simulink model "Part11_Unreal_Engine"  (R2021a)
settings: Solver=VariableStepAuto  StartTime=0.0  StopTime=100  RelTol=1e-3
libraries: vdynlib x3, vrlib x2, simulink x2, sim3dlib x1, mpcadaslib x1, pid_lib x1
settings Model: Creator=QZHAN112  LastModifiedBy=QZHAN112

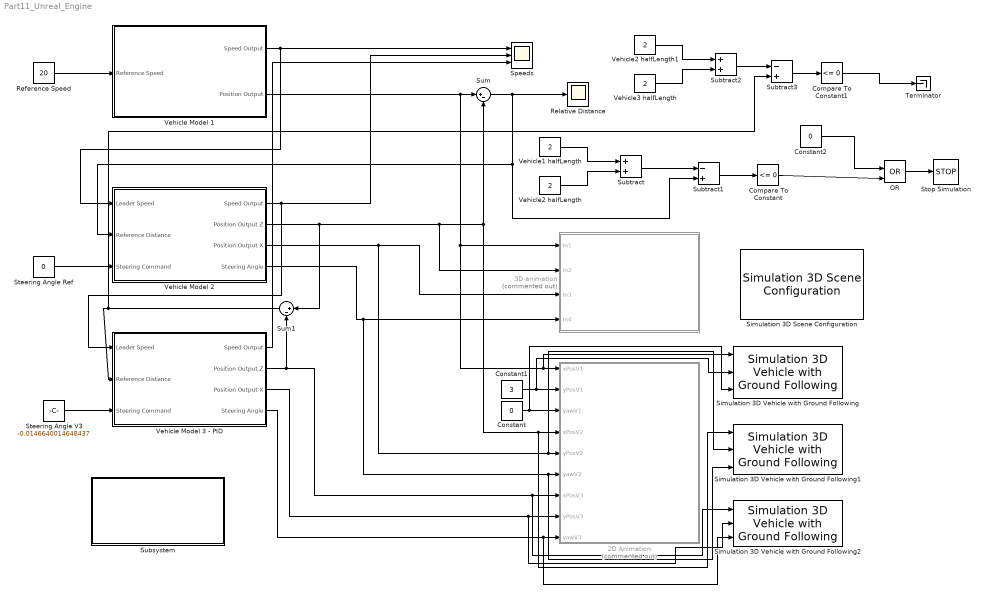
== system Part11_Unreal_Engine ==
  2D Animation : Subsystem  Commented=on
  3D animation : Subsystem  Commented=on
  Compare To Constant : simulink/Logic and Bit Operations/Compare To Constant  relop=<=  const=0  OutDataTypeStr=boolean
  Compare To Constant1 : simulink/Logic and Bit Operations/Compare To Constant  relop=<=  const=0  OutDataTypeStr=boolean
  Constant : Constant  Value=0
  Constant1 : Constant  Value=3
  Constant2 : Constant  Value=0
  OR : Logic  Operator=OR  IconShape=distinctive  AllPortsSameDT=off  OutDataTypeStr=boolean
  Reference Speed : Constant  Value=20
  Relative Distance : Scope
  Simulation 3D Scene Configuration : sim3dlib/Simulation 3D Scene Configuration  Priority=0  ProjectFormat=Default Scenes  SceneDesc=Straight road  ProjectName=C:\Program Files\MATLAB\R2021a\toolbox\shared\sim3d_projects\automotive_project\UE4\WindowsNoEditor\VehicleSimulation.exe  ScenePath=/Game/Maps/HwStrght  vehTagList={'Scene Origin';'SimulinkVehicle1';'SimulinkVehicle2';'SimulinkVehicle3'}  vehTag=SimulinkVehicle2  OpVisEn=off  Ts=0.1  EnableWindow=on  EnableWeather=off  SunAltitude=40.0  SunAzimuth=90  clouds=10  wind=1  fog=0  rain=0  sensorTag=MainCamera1  sensorId=1  sensorName=MainCamera1  mountLoc=Origin  offsetFlag=off  tmountOffset=[0, 0, 0]  rmountOffset=[0, 0, 0]  HorizontalResolution=1280  VerticalResolution=720  HorizontalFOV=60  mountPoint=[0 0 0]  mountOrientation=[0 0 0]  aMode=3  ID=1
      settings: SourceProductBaseCode=DR,UV,VE
  Simulation 3D Vehicle with Ground Following : vdynlib/Vehicle Scenarios/Sim3D/Sim3D Vehicle/Components/Simulation 3D Vehicle with Ground Following  Priority=-1  PassVehMesh=Small pickup truck  MeshPath=/MathWorksSimulation/Vehicles/Muscle/Meshes/SK_MuscleCar.SK_MuscleCar  TrackWidth=1.9  WheelBase=3  WheelRadius=0.35  VehColor=Red  InitialPos=[40, 0, 0]  InitialRot=[0, 0, 0]  ActorName=SimulinkVehicle1  VehLightsControl=off  HeadlightColor=[ 1, 1, 1 ]  HighBeamIntensity=100000  LowBeamIntensity=60000  HighBeamConeAngle=1.22  LowBeamConeAngle=1.22  LeftHeadlightOrientation=[ 0, 0 ]  RightHeadlightOrientation=[ 0, 0 ]  BrakelightIntensity=200  ReverselightIntensity=500  SignallightIntensity=500  SignallightPeriod=1  SignalPulseWidth=50  SampleTime=0.1  ActorType=SimulinkVehicle  ID=1  aMode=2  ActorTag=SimulinkVehicle1  CoordinateScheme=SAE
      settings: SourceProductBaseCode=VE
  Simulation 3D Vehicle with Ground Following1 : vdynlib/Vehicle Scenarios/Sim3D/Sim3D Vehicle/Components/Simulation 3D Vehicle with Ground Following  Priority=-1  PassVehMesh=Sedan  MeshPath=/MathWorksSimulation/Vehicles/Muscle/Meshes/SK_MuscleCar.SK_MuscleCar  TrackWidth=1.9  WheelBase=3  WheelRadius=0.35  VehColor=Silver  InitialPos=[20, 0, 0]  InitialRot=[0, 0, 0]  ActorName=SimulinkVehicle2  VehLightsControl=off  HeadlightColor=[ 1, 1, 1 ]  HighBeamIntensity=100000  LowBeamIntensity=60000  HighBeamConeAngle=1.22  LowBeamConeAngle=1.22  LeftHeadlightOrientation=[ 0, 0 ]  RightHeadlightOrientation=[ 0, 0 ]  BrakelightIntensity=200  ReverselightIntensity=500  SignallightIntensity=500  SignallightPeriod=1  SignalPulseWidth=50  SampleTime=0.1  ActorType=SimulinkVehicle  ID=2  aMode=2  ActorTag=SimulinkVehicle2  CoordinateScheme=SAE
      settings: SourceProductBaseCode=VE
  Simulation 3D Vehicle with Ground Following2 : vdynlib/Vehicle Scenarios/Sim3D/Sim3D Vehicle/Components/Simulation 3D Vehicle with Ground Following  Priority=-1  PassVehMesh=Box truck  MeshPath=/MathWorksSimulation/Vehicles/Muscle/Meshes/SK_MuscleCar.SK_MuscleCar  TrackWidth=1.9  WheelBase=3  WheelRadius=0.35  VehColor=Green  InitialPos=[0, 100, 0]  InitialRot=[0, 0, 0]  ActorName=SimulinkVehicle3  VehLightsControl=off  HeadlightColor=[ 1, 1, 1 ]  HighBeamIntensity=100000  LowBeamIntensity=60000  HighBeamConeAngle=1.22  LowBeamConeAngle=1.22  LeftHeadlightOrientation=[ 0, 0 ]  RightHeadlightOrientation=[ 0, 0 ]  BrakelightIntensity=200  ReverselightIntensity=500  SignallightIntensity=500  SignallightPeriod=1  SignalPulseWidth=50  SampleTime=0.1  ActorType=SimulinkVehicle  ID=3  aMode=2  ActorTag=SimulinkVehicle3  CoordinateScheme=SAE
      settings: SourceProductBaseCode=VE
  Speeds : Scope  NumInputPorts=3
  Steering Angle Ref : Constant  Value=0
  Steering Angle V3 : Constant  Value=-0.0146640014648437
  Stop Simulation : Stop
  Subsystem : Subsystem
  Subtract : Sum
  Subtract1 : Sum  Inputs=-+
  Subtract2 : Sum
  Subtract3 : Sum  Inputs=-+
  Sum : Sum  Inputs=|+-
  Sum1 : Sum  Inputs=|+-
  Terminator : Terminator
  Vehicle Model 1 : Subsystem  mask{Pos=40, Speed=20}
      mask prompts: Pos "Initial Position"; Speed "Initial Speed"
      mask TypeOptions Pos: Initial Position/Value
      mask TypeOptions Speed: Initial Speed/Value
      mask Display: image('model-based autonomous traffic simulation framework\Scratch.jpg');
  Vehicle Model 2 : Subsystem  mask{Pos=20, Speed=25}
      mask prompts: Pos "Initial Position"; Speed "Initial Speed"
      mask TypeOptions Pos: Initial Position Z/Value
      mask TypeOptions Speed: Initial Speed/Value
      mask Display: image('model-based autonomous traffic simulation framework\Car-Design-Drawing-From-Shoulder.jpg');
  Vehicle Model 3 - PID : Subsystem  mask{Pos=0, Speed=20}
      mask prompts: Pos "Initial Position"; Speed "Initial Speed"
      mask TypeOptions Pos: Initial Position Z/Value
      mask TypeOptions Speed: Initial Speed/Value
      mask Display: image('model-based autonomous traffic simulation framework\Caton.jpg');
  Vehicle1 halfLength : Constant  Value=2
  Vehicle2 halfLength : Constant  Value=2
  Vehicle2 halfLength1 : Constant  Value=2
  Vehicle3 halfLength : Constant  Value=2
  wires:
  Vehicle Model 1/2(Position Output) -> Simulation 3D Vehicle with Ground Following/1, 2D Animation/1(xPosV1), 3D animation/1(In1), Sum/1
  Reference Speed/1 -> Vehicle Model 1/1(Reference Speed)
  Vehicle Model 2/1(Speed Output) -> Vehicle Model 3 - PID/1(Leader Speed), Speeds/2
  Vehicle Model 1/1(Speed Output) -> Speeds/1, Vehicle Model 2/1(Leader Speed)
  Sum/1 -> Relative Distance/1, Vehicle Model 2/2(Reference Distance), Subtract1/2
  Vehicle Model 2/2(Position Output Z) -> Sum1/1, Simulation 3D Vehicle with Ground Following1/1, 2D Animation/4(xPosV2), Sum/2, 3D animation/2(In2)
  Steering Angle Ref/1 -> Vehicle Model 2/3(Steering Command)
  Vehicle Model 2/3(Position Output X) -> Simulation 3D Vehicle with Ground Following1/2, 2D Animation/5(yPosV2), 3D animation/3(In3)
  Vehicle Model 2/4(Steering Angle) -> Simulation 3D Vehicle with Ground Following1/3, 2D Animation/6(yawV2), 3D animation/4(In4)
  Constant/1 -> Simulation 3D Vehicle with Ground Following/3, 2D Animation/3(yawV1)
  Constant1/1 -> Simulation 3D Vehicle with Ground Following/2, 2D Animation/2(yPosV1)
  Vehicle1 halfLength/1 -> Subtract/1
  Vehicle2 halfLength/1 -> Subtract/2
  Subtract/1 -> Subtract1/1
  Subtract1/1 -> Compare To Constant/1
  Vehicle Model 3 - PID/2(Position Output Z) -> Simulation 3D Vehicle with Ground Following2/1, 2D Animation/7(xPosV3), Sum1/2
  Vehicle Model 3 - PID/3(Position Output X) -> Simulation 3D Vehicle with Ground Following2/2, 2D Animation/8(yPosV3)
  Vehicle Model 3 - PID/4(Steering Angle) -> Simulation 3D Vehicle with Ground Following2/3, 2D Animation/9(yawV3)
  Sum1/1 -> Vehicle Model 3 - PID/2(Reference Distance), Subtract3/2
  Vehicle Model 3 - PID/1(Speed Output) -> Speeds/3
  Vehicle3 halfLength/1 -> Subtract2/2
  Vehicle2 halfLength1/1 -> Subtract2/1
  Subtract2/1 -> Subtract3/1
  Subtract3/1 -> Compare To Constant1/1
  OR/1 -> Stop Simulation/1
  Compare To Constant/1 -> OR/2
  Compare To Constant1/1 -> Terminator/1
  Constant2/1 -> OR/1
  Steering Angle V3/1 -> Vehicle Model 3 - PID/3(Steering Command)

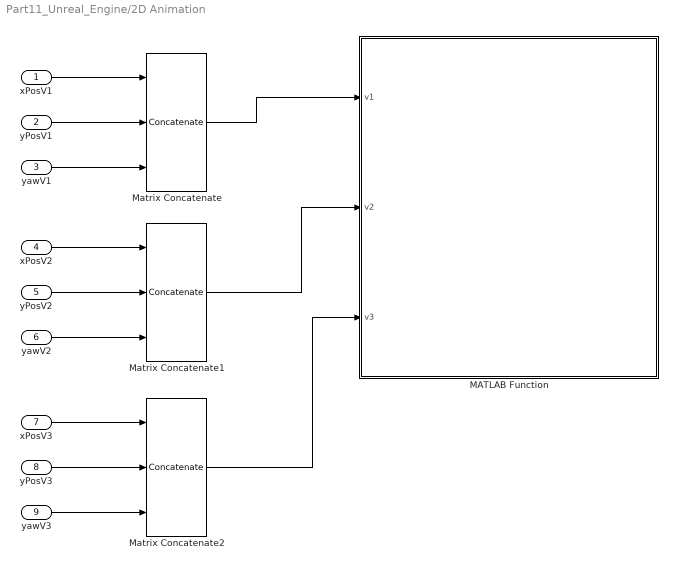
== system Part11_Unreal_Engine/2D Animation ==
  xPosV1 : Inport
  yPosV1 : Inport  Port=2
  yawV1 : Inport  Port=3
  xPosV2 : Inport  Port=4
  yPosV2 : Inport  Port=5
  yawV2 : Inport  Port=6
  xPosV3 : Inport  Port=7
  yPosV3 : Inport  Port=8
  yawV3 : Inport  Port=9
  MATLAB Function : MATLAB Function  TreatAsAtomicUnit=on
      mask init:
      | close all;
      | figure('units','normalized','outerposition',[0 0 1 1]);
      | % grid on
      | axis equal;
      | hold on
  Matrix Concatenate : Concatenate  NumInputs=3  ConcatenateDimension=2
  Matrix Concatenate1 : Concatenate  NumInputs=3  ConcatenateDimension=2
  Matrix Concatenate2 : Concatenate  NumInputs=3  ConcatenateDimension=2
  wires:
  Matrix Concatenate/1 -> MATLAB Function/1(v1)
  yawV1/1 -> Matrix Concatenate/3
  yPosV1/1 -> Matrix Concatenate/2
  xPosV1/1 -> Matrix Concatenate/1
  xPosV2/1 -> Matrix Concatenate1/1
  yPosV2/1 -> Matrix Concatenate1/2
  yawV2/1 -> Matrix Concatenate1/3
  Matrix Concatenate1/1 -> MATLAB Function/2(v2)
  Matrix Concatenate2/1 -> MATLAB Function/3(v3)
  yawV3/1 -> Matrix Concatenate2/3
  yPosV3/1 -> Matrix Concatenate2/2
  xPosV3/1 -> Matrix Concatenate2/1

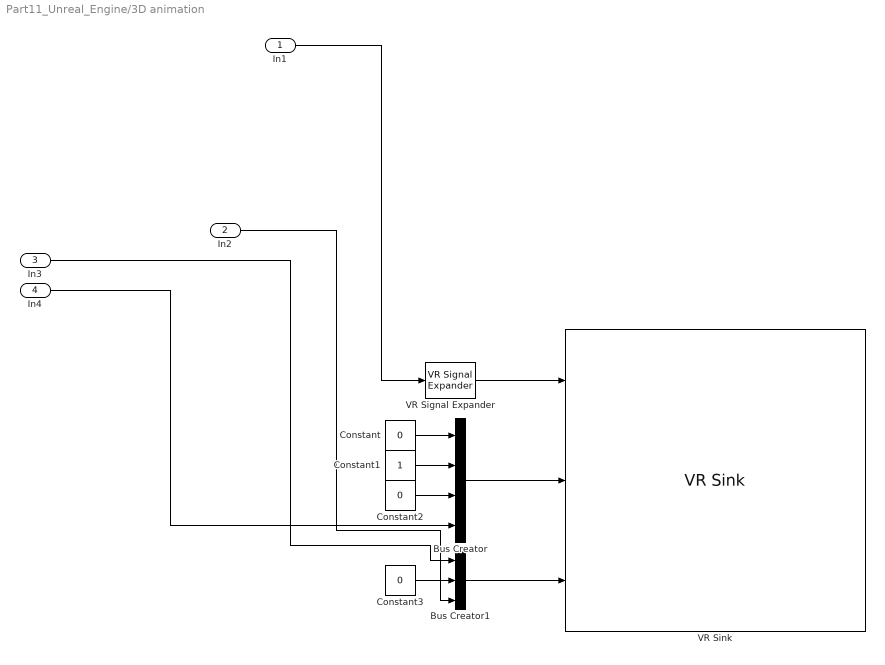
== system Part11_Unreal_Engine/3D animation ==
  In1 : Inport
  In2 : Inport  Port=2
  In3 : Inport  Port=3
  In4 : Inport  Port=4
  Bus Creator : BusCreator  Inputs=4
  Bus Creator1 : BusCreator  Inputs=3
  Constant : Constant  Value=0
  Constant1 : Constant
  Constant2 : Constant  Value=0
  Constant3 : Constant  Value=0
  VR Signal Expander : vrlib/VR Signal Expander  outwidth=3  outidx=[3]
  VR Sink : vrlib/VR Sink  InstantiateOnLoad=on  SampleTime=1  ViewEnable=on  RemoteChange=off  RemoteView=off  FieldsWritten=Car_Red.translation.3.1.1.double#Car_Blue.rotation.4.1.1.double#Car_Blue.translation.3.1.1.double  WorldFileName=PlatoonWorld.WRL  AutoView=off  VideoDimensions=[]  AllowVariableSize=off
  wires:
  Bus Creator1/1 -> VR Sink/3
  Constant1/1 -> Bus Creator/2
  VR Signal Expander/1 -> VR Sink/1
  Constant2/1 -> Bus Creator/3
  Constant/1 -> Bus Creator/1
  Bus Creator/1 -> VR Sink/2
  Constant3/1 -> Bus Creator1/2
  In3/1 -> Bus Creator1/1
  In4/1 -> Bus Creator/4
  In1/1 -> VR Signal Expander/1
  In2/1 -> Bus Creator1/3

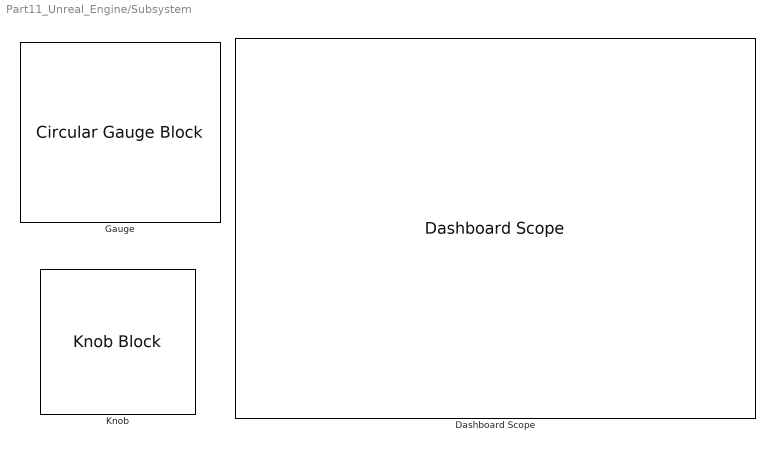
== system Part11_Unreal_Engine/Subsystem ==
  Dashboard Scope : DashboardScope
  Gauge : CircularGaugeBlock
  Knob : KnobBlock  ScaleMin=-1  ScaleMax=1

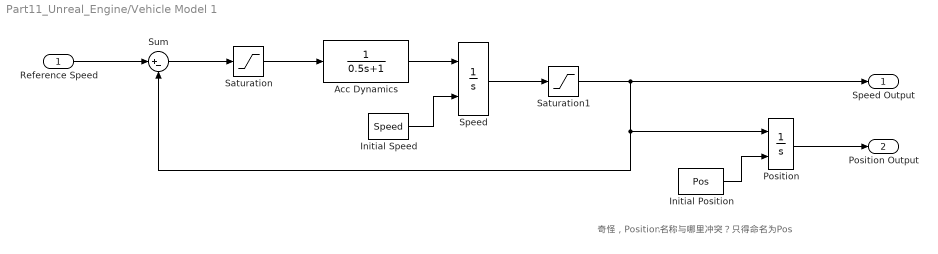
== system Part11_Unreal_Engine/Vehicle Model 1 ==
  note: 奇怪，Position名称与哪里冲突？只得命名为Pos
  Reference Speed : Inport
  Acc Dynamics : TransferFcn  Denominator=[0.5 1]
  Initial Position : Constant  Value=Pos
  Initial Speed : Constant  Value=Speed
  Position : Integrator  InitialConditionSource=external
  Saturation : Saturate  UpperLimit=2  LowerLimit=-3
  Saturation1 : Saturate  UpperLimit=inf  LowerLimit=0
  Speed : Integrator  InitialConditionSource=external
  Sum : Sum  Inputs=|+-
  Speed Output : Outport
  Position Output : Outport  Port=2
  wires:
  Saturation/1 -> Acc Dynamics/1
  Acc Dynamics/1 -> Speed/1
  Speed/1 -> Saturation1/1
  Position/1 -> Position Output/1
  Saturation1/1 -> Speed Output/1, Sum/2, Position/1
  Reference Speed/1 -> Sum/1
  Initial Speed/1 -> Speed/2
  Sum/1 -> Saturation/1
  Initial Position/1 -> Position/2

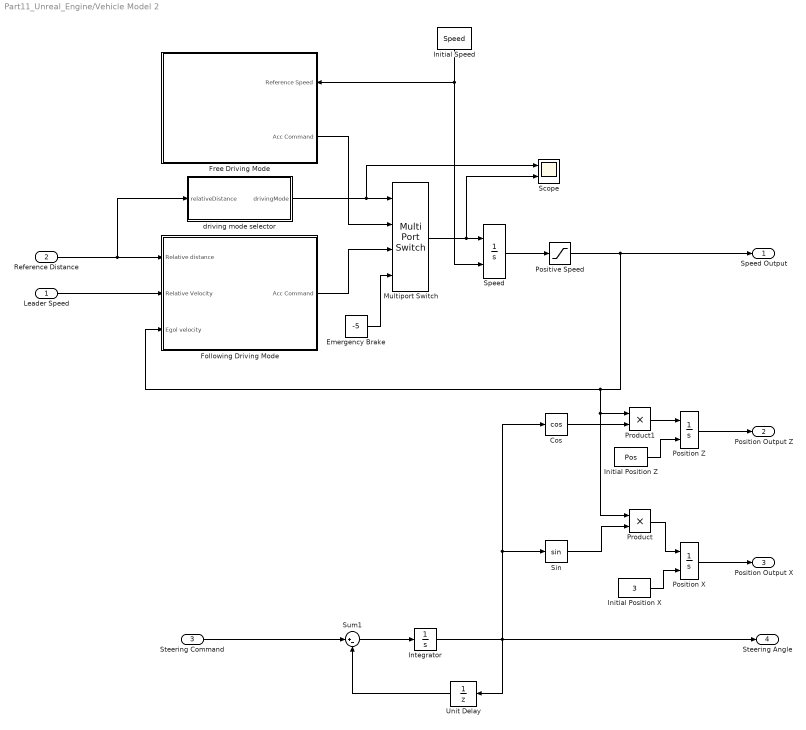
== system Part11_Unreal_Engine/Vehicle Model 2 ==
  Leader Speed : Inport
  Reference Distance : Inport  Port=2
  Steering Command : Inport  Port=3
  Cos : Trigonometry  Operator=cos
  Emergency Brake : Constant  Value=-5
  Following Driving Mode : Subsystem
  Free Driving Mode : Subsystem
      settings: PortSchema="{\"entries\":[{\"content\":{\"sides\":[{\"content\":{\"connectorIds\":[]},\"type\":\"ConnectorPlacement.EquallySpacedRectSide\",\"uuid\":\"610b25c5-b833-48d8-91de-4e4522f1e869\"},{\"content\":{\"connectorIds\":[\"In1\",\"Out1\"],\"side\":\"RIGHT\"},\"type\":\"ConnectorPlacement.EquallySpacedRectSide\",\"uuid\":\"bfbfafdf-9638-4c83-9a6c-a30c0fb24eff\"},{\"content\":{\"connectorIds\":[],\"side\":\"TOP\"},\"type\":\"ConnectorPlacement.EquallySpacedRectSide\",\"uuid\":\"2708cd9c-977e-4237-a5bd-2827f533dc12\"}]},\"type\":\"ConnectorPlacement.EquallySpacedConnector\",\"uuid\":\"23ea83fe-0fb5-46b9-9450-330af3b093f3\"}],\"packageUris\":[\"http://schema.mathworks.com/mf0/Connector/R2020b\"],\"version\":\"1.0\"}"
  Initial Position X : Constant  Value=3
  Initial Position Z : Constant  Value=Pos
  Initial Speed : Constant  Value=Speed
  Integrator : Integrator
  Multiport Switch : MultiPortSwitch
  Position X : Integrator  InitialConditionSource=external
  Position Z : Integrator  InitialConditionSource=external
  Positive Speed : Saturate  UpperLimit=inf  LowerLimit=0
  Product : Product
  Product1 : Product
  Scope : Scope  NumInputPorts=2
  Sin : Trigonometry
  Speed : Integrator  InitialConditionSource=external
  Sum1 : Sum  Inputs=|+-
  Unit Delay : UnitDelay  SampleTime=-1  HasFrameUpgradeWarning=on
  driving mode selector : Stateflow chart  TreatAsAtomicUnit=on
  Speed Output : Outport
  Position Output Z : Outport  Port=2
  Position Output X : Outport  Port=3
  Steering Angle : Outport  Port=4
  wires:
  Speed/1 -> Positive Speed/1
  Position Z/1 -> Position Output Z/1
  Initial Speed/1 -> Speed/2, Free Driving Mode/1(Reference Speed)
  Initial Position Z/1 -> Position Z/2
  Positive Speed/1 -> Speed Output/1, Following Driving Mode/3(Egol velocity), Product/1, Product1/1
  Sum1/1 -> Integrator/1
  Steering Command/1 -> Sum1/1
  Integrator/1 -> Steering Angle/1, Cos/1, Sin/1, Unit Delay/1
  Unit Delay/1 -> Sum1/2
  Sin/1 -> Product/2
  Initial Position X/1 -> Position X/2
  Position X/1 -> Position Output X/1
  Product/1 -> Position X/1
  Cos/1 -> Product1/2
  Product1/1 -> Position Z/1
  Reference Distance/1 -> driving mode selector/1(relativeDistance), Following Driving Mode/1(Relative distance)
  Leader Speed/1 -> Following Driving Mode/2(Relative Velocity)
  Following Driving Mode/1(Acc Command) -> Multiport Switch/3
  Free Driving Mode/1(Acc Command) -> Multiport Switch/2
  Multiport Switch/1 -> Scope/2, Speed/1
  Emergency Brake/1 -> Multiport Switch/4
  driving mode selector/1(drivingMode) -> Scope/1, Multiport Switch/1

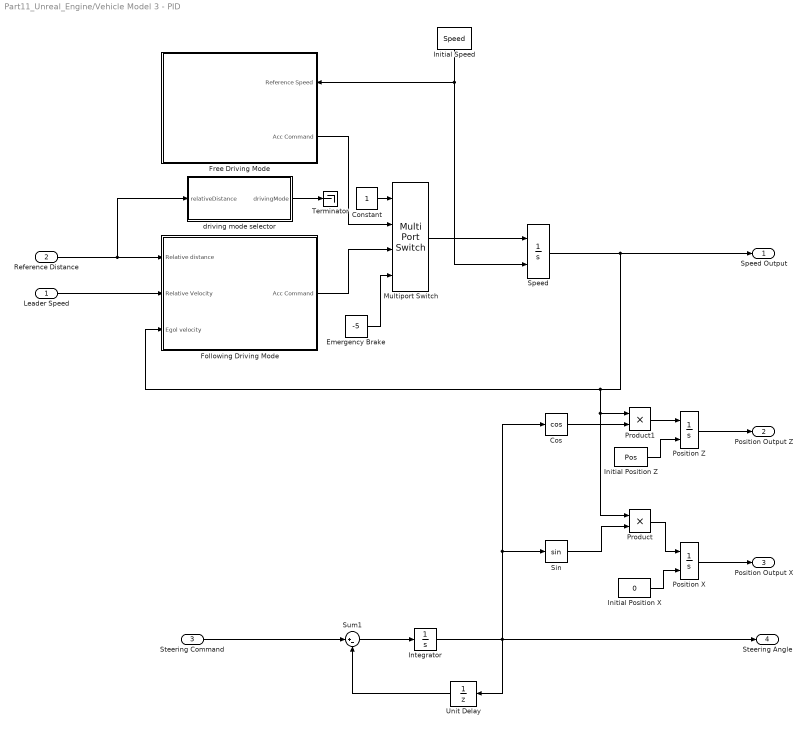
== system Part11_Unreal_Engine/Vehicle Model 3 - PID ==
  Leader Speed : Inport
  Reference Distance : Inport  Port=2
  Steering Command : Inport  Port=3
  Constant : Constant
  Cos : Trigonometry  Operator=cos
  Emergency Brake : Constant  Value=-5
  Following Driving Mode : Subsystem
  Free Driving Mode : Subsystem
      settings: PortSchema="{\"entries\":[{\"content\":{\"sides\":[{\"content\":{\"connectorIds\":[]},\"type\":\"ConnectorPlacement.EquallySpacedRectSide\",\"uuid\":\"610b25c5-b833-48d8-91de-4e4522f1e869\"},{\"content\":{\"connectorIds\":[\"In1\",\"Out1\"],\"side\":\"RIGHT\"},\"type\":\"ConnectorPlacement.EquallySpacedRectSide\",\"uuid\":\"bfbfafdf-9638-4c83-9a6c-a30c0fb24eff\"},{\"content\":{\"connectorIds\":[],\"side\":\"TOP\"},\"type\":\"ConnectorPlacement.EquallySpacedRectSide\",\"uuid\":\"2708cd9c-977e-4237-a5bd-2827f533dc12\"}]},\"type\":\"ConnectorPlacement.EquallySpacedConnector\",\"uuid\":\"23ea83fe-0fb5-46b9-9450-330af3b093f3\"}],\"packageUris\":[\"http://schema.mathworks.com/mf0/Connector/R2020b\"],\"version\":\"1.0\"}"
  Initial Position X : Constant  Value=0
  Initial Position Z : Constant  Value=Pos
  Initial Speed : Constant  Value=Speed
  Integrator : Integrator
  Multiport Switch : MultiPortSwitch
  Position X : Integrator  InitialConditionSource=external
  Position Z : Integrator  InitialConditionSource=external
  Product : Product
  Product1 : Product
  Sin : Trigonometry
  Speed : Integrator  InitialConditionSource=external  LimitOutput=on  LowerSaturationLimit=0
  Sum1 : Sum  Inputs=|+-
  Terminator : Terminator
  Unit Delay : UnitDelay  SampleTime=-1  HasFrameUpgradeWarning=on
  driving mode selector : Stateflow chart  TreatAsAtomicUnit=on
  Speed Output : Outport
  Position Output Z : Outport  Port=2
  Position Output X : Outport  Port=3
  Steering Angle : Outport  Port=4
  wires:
  driving mode selector/1(drivingMode) -> Terminator/1
  Emergency Brake/1 -> Multiport Switch/4
  Multiport Switch/1 -> Speed/1
  Free Driving Mode/1(Acc Command) -> Multiport Switch/2
  Following Driving Mode/1(Acc Command) -> Multiport Switch/3
  Leader Speed/1 -> Following Driving Mode/2(Relative Velocity)
  Reference Distance/1 -> Following Driving Mode/1(Relative distance), driving mode selector/1(relativeDistance)
  Product1/1 -> Position Z/1
  Cos/1 -> Product1/2
  Product/1 -> Position X/1
  Position X/1 -> Position Output X/1
  Initial Position X/1 -> Position X/2
  Sin/1 -> Product/2
  Unit Delay/1 -> Sum1/2
  Integrator/1 -> Unit Delay/1, Sin/1, Cos/1, Steering Angle/1
  Steering Command/1 -> Sum1/1
  Sum1/1 -> Integrator/1
  Speed/1 -> Product1/1, Product/1, Following Driving Mode/3(Egol velocity), Speed Output/1
  Initial Position Z/1 -> Position Z/2
  Initial Speed/1 -> Free Driving Mode/1(Reference Speed), Speed/2
  Position Z/1 -> Position Output Z/1
  Constant/1 -> Multiport Switch/1

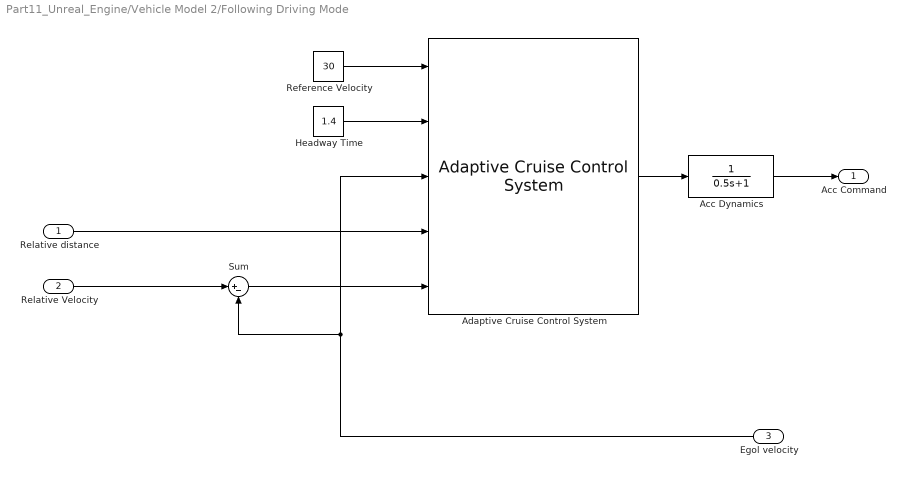
== system Part11_Unreal_Engine/Vehicle Model 2/Following Driving Mode ==
  Relative distance : Inport
  Relative Velocity : Inport  Port=2
  Egol velocity : Inport  Port=3
  Acc Dynamics : TransferFcn  Denominator=[0.5 1]
  Adaptive Cruise Control System : mpcadaslib/Adaptive Cruise Control System  EgoModel=tf(1,[0.5,1,0])  InitialEgoVelocity=30  DefaultSpacing=10  MaxVelocity=50  MinAcceleration=-3  amin_ext=off  MaxAcceleration=2  amax_ext=off  Ts=0.02  PredictionHorizon=300  ControllerBehavior=0.800  suboptimal=off  maxiter=10  datatypeopt=double  optmode=off  trackmode=off
  Headway Time : Constant  Value=1.4
  Reference Velocity : Constant  Value=30
  Sum : Sum  Inputs=|+-
  Acc Command : Outport
  wires:
  Adaptive Cruise Control System/1 -> Acc Dynamics/1
  Sum/1 -> Adaptive Cruise Control System/5
  Reference Velocity/1 -> Adaptive Cruise Control System/1
  Relative distance/1 -> Adaptive Cruise Control System/4
  Egol velocity/1 -> Adaptive Cruise Control System/3, Sum/2
  Relative Velocity/1 -> Sum/1
  Headway Time/1 -> Adaptive Cruise Control System/2
  Acc Dynamics/1 -> Acc Command/1

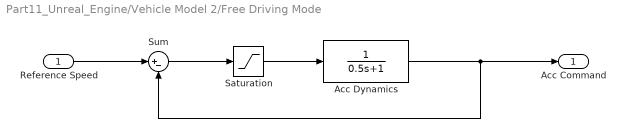
== system Part11_Unreal_Engine/Vehicle Model 2/Free Driving Mode ==
  Reference Speed : Inport
  Acc Dynamics : TransferFcn  Denominator=[0.5 1]
  Saturation : Saturate  UpperLimit=2  LowerLimit=-3
  Sum : Sum  Inputs=|+-
  Acc Command : Outport
  wires:
  Saturation/1 -> Acc Dynamics/1
  Acc Dynamics/1 -> Sum/2, Acc Command/1
  Sum/1 -> Saturation/1
  Reference Speed/1 -> Sum/1

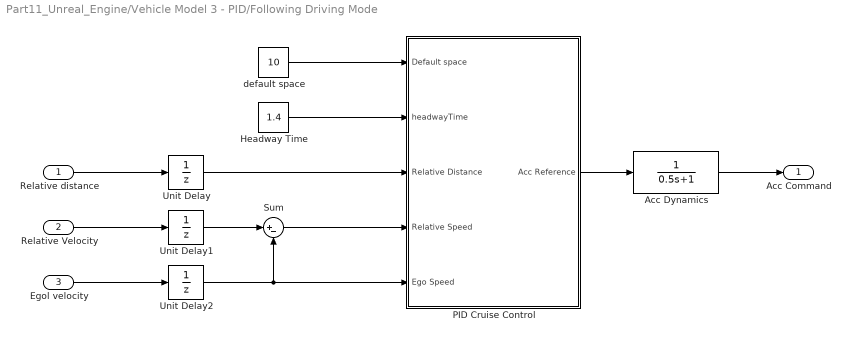
== system Part11_Unreal_Engine/Vehicle Model 3 - PID/Following Driving Mode ==
  Relative distance : Inport
  Relative Velocity : Inport  Port=2
  Egol velocity : Inport  Port=3
  Acc Dynamics : TransferFcn  Denominator=[0.5 1]
  Headway Time : Constant  Value=1.4
  PID Cruise Control : Subsystem
  Sum : Sum  Inputs=|+-
  Unit Delay : UnitDelay  SampleTime=-1  HasFrameUpgradeWarning=on
  Unit Delay1 : UnitDelay  SampleTime=-1  HasFrameUpgradeWarning=on
  Unit Delay2 : UnitDelay  SampleTime=-1  HasFrameUpgradeWarning=on
  default space : Constant  Value=10
  Acc Command : Outport
  wires:
  Acc Dynamics/1 -> Acc Command/1
  Headway Time/1 -> PID Cruise Control/2(headwayTime)
  Relative Velocity/1 -> Unit Delay1/1
  Egol velocity/1 -> Unit Delay2/1
  Relative distance/1 -> Unit Delay/1
  default space/1 -> PID Cruise Control/1(Default space)
  Sum/1 -> PID Cruise Control/4(Relative Speed)
  PID Cruise Control/1(Acc Reference) -> Acc Dynamics/1
  Unit Delay/1 -> PID Cruise Control/3(Relative Distance)
  Unit Delay1/1 -> Sum/1
  Unit Delay2/1 -> PID Cruise Control/5(Ego Speed), Sum/2

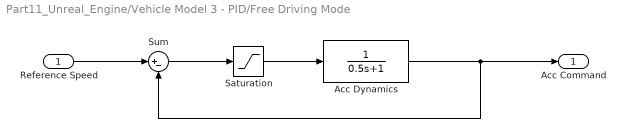
== system Part11_Unreal_Engine/Vehicle Model 3 - PID/Free Driving Mode ==
  Reference Speed : Inport
  Acc Dynamics : TransferFcn  Denominator=[0.5 1]
  Saturation : Saturate  UpperLimit=2  LowerLimit=-3
  Sum : Sum  Inputs=|+-
  Acc Command : Outport
  wires:
  Reference Speed/1 -> Sum/1
  Sum/1 -> Saturation/1
  Acc Dynamics/1 -> Acc Command/1, Sum/2
  Saturation/1 -> Acc Dynamics/1

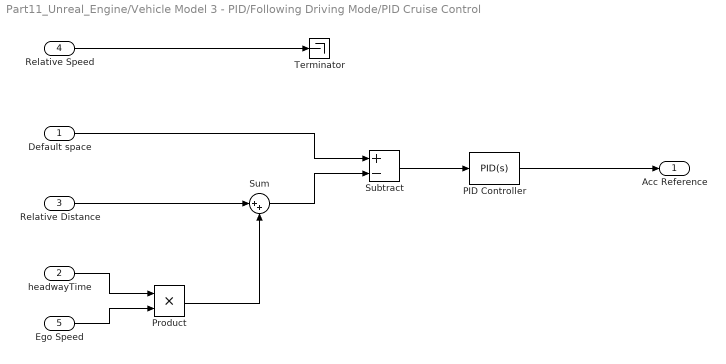
== system Part11_Unreal_Engine/Vehicle Model 3 - PID/Following Driving Mode/PID Cruise Control ==
  Default space : Inport
  headwayTime : Inport  Port=2
  Relative Distance : Inport  Port=3
  Relative Speed : Inport  Port=4
  Ego Speed : Inport  Port=5
  PID Controller : pid_lib/PID Controller  Controller=PID  Form=Parallel  TimeDomain=Continuous-time  UseExternalTs=off  SampleTime=-1  IntegratorMethod=Forward Euler  FilterMethod=Forward Euler  ControllerParametersSource=internal  P=2  I=0.04  D=2.1  UseFilter=on  N=230  TunerSelectOption=Transfer Function Based (PID Tuner App)  InitialConditionSource=internal  InitialConditionForIntegrator=0  InitialConditionForFilter=0  DifferentiatorICPrevScaledInput=0  ExternalReset=none  TrackingMode=off  Kt=1  LimitOutput=on  SatLimitsSource=internal  UpperSaturationLimit=2  LowerSaturationLimit=-3  LinearizeAsGain=on  AntiWindupMode=clamping  Kb=1  POutMin=[]  POutMax=[]  IOutMin=[]  IOutMax=[]  DOutMin=[]  DOutMax=[]  NOutMin=[]  NOutMax=[]  SumOutMin=[]  SumOutMax=[]  SaturationOutMin=[]  SaturationOutMax=[]  PParamMin=[]  PParamMax=[]  IParamMin=[]  IParamMax=[]  DParamMin=[]  DParamMax=[]  NParamMin=[]  NParamMax=[]  KbParamMin=[]  KbParamMax=[]  KtParamMin=[]  KtParamMax=[]  KbOutMin=[]  KbOutMax=[]  KtOutMin=[]  KtOutMax=[]  IntegratorOutMin=[]  IntegratorOutMax=[]  FilterOutMin=[]  FilterOutMax=[]  SumI1OutMin=[]  SumI1OutMax=[]  SumI2OutMin=[]  SumI2OutMax=[]  SumI3OutMin=[]  SumI3OutMax=[]  SumI4OutMin=[]  SumI4OutMax=[]  SumDOutMin=[]  SumDOutMax=[]  DifferentiatorOutMin=[]  DifferentiatorOutMax=[]  FilterDiffOutCoefMin=[]  FilterDiffOutCoefMax=[]  ReciprocalOutMin=[]  ReciprocalOutMax=[]  SumDenOutMin=[]  SumDenOutMax=[]  SumNumOutMin=[]  SumNumOutMax=[]  DivideOutMin=[]  DivideOutMax=[]  UdiffTsProdOutMin=[]  UdiffTsProdOutMax=[]  NTsProdOutMin=[]  NTsProdOutMax=[]  UintegralTsProdOutMin=[]  UintegralTsProdOutMax=[]  UngainTsProdOutMin=[]  UngainTsProdOutMax=[]  IntegratorContinuousStateAttributes=''  IntegratorStateMustResolveToSignalObject=off  IntegratorRTWStateStorageClass=Auto  FilterContinuousStateAttributes=''  FilterStateMustResolveToSignalObject=off  FilterRTWStateStorageClass=Auto  ParallelPVariant=InternalParameters  IdealPVariant=Disabled  IVariant=InternalParameters  DVariant=InternalParameters  IntegratorVariant=Continuous  SatVariant=Enabled  AWVariant=ContClampingParallel  PCopyVariant=Disabled  TRVariant=Disabled  FdbkBlocksVariant=Forward  IdealPFdbkVariant=Disabled  SatFdbkVariant=Disabled  DerivativeFilterVariant=ContFilter  NVariant=InternalParameters  NCopyVariant=Disabled  FilterICVariant=InternalICsFilter  IntegratorICVariant=InternalICs  ExternalResetVariant=Disabled  TRSumVariant=Passthrough  SumFdbkVariant=Disabled  SumVariant=Sum_PID  TsampFilterVariant=InternalTs  TsampNgainVariant=Passthrough  TsampIntegralVariant=Passthrough  ExternalSaturationOutDataTypeStr=Inherit: Same as second input
  Product : Product
  Subtract : Sum  Inputs=+-
  Sum : Sum  Inputs=|++
  Terminator : Terminator
  Acc Reference : Outport
  wires:
  headwayTime/1 -> Product/1
  Ego Speed/1 -> Product/2
  Relative Distance/1 -> Sum/1
  Product/1 -> Sum/2
  Sum/1 -> Subtract/2
  Default space/1 -> Subtract/1
  Subtract/1 -> PID Controller/1
  PID Controller/1 -> Acc Reference/1
  Relative Speed/1 -> Terminator/1

== stateflow chart Part11_Unreal_Engine/Vehicle Model 2/driving mode selector ==
  state FollowingMode
    entry:
    drivingMode = 2;
  state FreeMode
    entry:
    drivingMode = 1;
  state EmergencyBrake
    entry:
    drivingMode = 3;
  (default) -> FreeMode
  FollowingMode -> FreeMode [order 1] : [relativeDistance > 50]
  FreeMode -> FollowingMode [order 1] : [relativeDistance <= 40]
  FreeMode -> EmergencyBrake [order 2] : [relativeDistance <= 10]
  FollowingMode -> EmergencyBrake [order 2] : [relativeDistance <= 10]
  EmergencyBrake -> FollowingMode : [relativeDistance >= 15]
  data: drivingMode output; relativeDistance input

== matlab function Part11_Unreal_Engine/2D Animation/MATLAB Function ==
  data: v1 input; v2 input; v3 input
function plotVehicle(v1, v2, v3)

% Clear previous vehicle
cla;

for v=[v1, v2, v3]

    x = v(1);
    y = v(2);
    yaw = v(3);

    centerP = [x; y];
    halflength_v = 2;
    halfwidth_v = 1;

    % Create a retangle represent a vehicle
    p1 = [ halflength_v;  halfwidth_v];
    p2 = [ halflength_v; -halfwidth_v];
    p3 = [-halflength_v; -halfwidth_v];
    p4 = [-halflength_v;  halfwidth_v];

    % Rotation Matrix
    rotatrix = [cos(yaw) -sin(yaw); sin(yaw) cos(yaw)];

    % Rotated Points
    % 这里用极坐标的参数方程来推导，然后用矩阵和向量的乘法
    % x = rcosθ     
    % y = rsinθ
    % x' = rcos(θ + A) => r(cosθcosA - sinθsinA) => rcosθcosA - rsinθsinA
    %                                            => xcosA - ysinA
    % y' = rsin(θ + A) => r(sinθcosA + cosθsinA) => rsinθcosA + rcosθsinA
    %                                            => ycosA + xsinA
    % 
    % |cosA -sinA| |x|       |xcosA - ysinA|
    % |sinA  cosA| |y|   =>  |xsinA + ycosA|
    %
    p1r = centerP + rotatrix*p1;
    p2r = centerP + rotatrix*p2;
    p3r = centerP + rotatrix*p3;
    p4r = centerP + rotatrix*p4;

    
    % Connecting points
    Hitbox = [p1r p2r p3r p4r p1r];


    % 将5个点的x坐标转化为一个列向量，y也一样
    cornersV_x = transpose(Hitbox(1,:));
    cornersV_y = transpose(Hitbox(2,:));
    
    
    % Plot vehicles
    if v == v1
        plot(cornersV_x,cornersV_y,'b'); % vehicel rectangle
        plot(x,y,'o'); % vehicle center
    elseif v == v2
        plot(cornersV_x,cornersV_y);
        plot(x,y);
    else
        plot(cornersV_x,cornersV_y,'g');
        plot(x,y,'*');
    end
    
end


% Plot road
upperline = plot([0 1000],[5 5],'color','#b0c4de','linewidth',4);
midLine = plot([0 1000],[0 0],'--','color','#b0c4de','linewidth',2);
lowerLine = plot([0 1000],[-5 -5],'color','#b0c4de','linewidth',4);


% Adjust axis
axis([x-50 x+50 y-20 y+20]);

== stateflow chart Part11_Unreal_Engine/Vehicle Model 3 - PID/driving mode selector ==
  state FollowingMode
    entry:
    drivingMode = 2;
  state FreeMode
    entry:
    drivingMode = 1;
  state EmergencyBrake
    entry:
    drivingMode = 3;
  (default) -> FreeMode
  FollowingMode -> FreeMode [order 1] : [relativeDistance > 60]
  FreeMode -> FollowingMode [order 1] : [relativeDistance <= 50]
  FreeMode -> EmergencyBrake [order 2] : [relativeDistance <= 25]
  FollowingMode -> EmergencyBrake [order 2] : [relativeDistance <= 25]
  EmergencyBrake -> FollowingMode : [relativeDistance >= 30]
  data: drivingMode output; relativeDistance input
